simulink model "m_robotic_phase"  (R2021b)
settings: Solver=ode4  StartTime=0.0  StopTime=tf  FixedStep=0.01  RelTol=1e-3
values from neighbouring files (symbols this model uses):
  X_init = 3*(rand(2,1)-0.5)    [PD_phase_robotic.m]    (also in phase_robotic.m = 2*(rand(2,1)-0.5))
  Xd_init = 3*(rand(2,1)-0.5)    [PD_phase_robotic.m]    (also in phase_robotic.m = 1*(rand(2,1)-0.5))
settings Model: Creator=Mando  LastModifiedBy=Mando

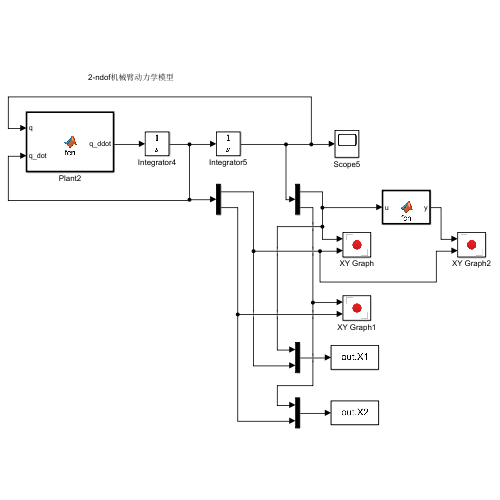
[thumbnail: Simulink's stored preview of the top-level diagram]
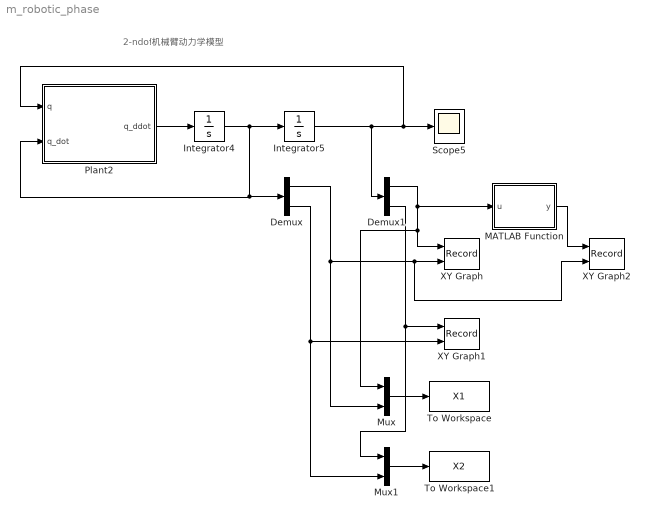
== system m_robotic_phase ==
  note: 2-ndof机械臂动力学模型
  Demux : Demux  Outputs=2
  Demux1 : Demux  Outputs=2
  Integrator4 : Integrator  InitialCondition=Xd_init
  Integrator5 : Integrator  InitialCondition=X_init
  MATLAB Function : MATLAB Function  TreatAsAtomicUnit=on
  Mux : Mux  Inputs=2
  Mux1 : Mux  Inputs=2
  Plant2 : MATLAB Function  TreatAsAtomicUnit=on
  Scope5 : Scope
  To Workspace : ToWorkspace  VariableName=X1  SampleTime=-1
  To Workspace1 : ToWorkspace  VariableName=X2  SampleTime=-1
  XY Graph : Record  FileSettingsInternal="{\"entries\":[{\"content\":{\"excelSettings\":{\"content\":{},\"type\":\"Streamout.ExcelSettings\"}},\"type\":\"Streamout.FileSettingStorage\",\"uuid\":\"9ba65a72-57f1-4f4d-8fe5-731dedb9ab80\"}],\"packageUris\":[\"http://schema.mathworks.com/mf0/streamout_blocks/R2020a\"],\"version\":\"1.0\"}"  Layout=[1 1]  SignalsInternal="{\"entries\":[{\"content\":{\"signals\":[{\"content\":{\"blockPath\":[\"m_robotic_phase/XY Graph\"],\"channel\":[],\"dimensions\":[1],\"domain\":\"m_robotic_phase/XY Graph\",\"lineColor\":\"#a2142f\",\"plots\":[1],\"port\":1,\"sid\":[\"\"],\"signalID\":74337,\"signalName\":\"Demux1:1\"},\"type\":\"RecordBlkView.Signal\",\"uuid\":\"b7ffe641-bfda-4282-85d4-15944fe21698\"},{\"content\":{\"blockPath\":[\"m_robotic_phase/XY Graph\"],\"channel\":[],\"dimensions\":[1],\"domain\":\"m_robotic_phase/XY Graph\",\"lineColor\":\"#139fff\",\"plots\":[1],\"port\":2,\"sid\":[\"\"],\"signalID\":74341,\"signalName\":\"Demux:1\"},\"type\":\"RecordBlkView.Signal\",\"uuid\":\"c2682a94-b715-47cb-b18e-efeff7ca8082\"}]},\"type\":\"RecordBlkView.InputSignals\",\"uuid\":\"df0cf377-e009-45f0-a3f5-9482d05fefdb\"}],\"packageUris\":[\"http://schema.mathworks.com/mf0/streamout_blocks/R2020a\"],\"version\":\"1.0\"}"  VisualizationBindings="{\"xyplotplugin\":{\"info\":[{\"series\":[{\"bindingParametersList\":[{\"parameter\":\"X-Axis\",\"signalID\":74337,\"signalName\":\"Demux1:1\"},{\"parameter\":\"Y-Axis\",\"signalID\":74341,\"signalName\":\"Demux:1\"}],\"seriesID\":17156}],\"subplotID\":1}]}}"  CompatibilityTag=XY
  XY Graph1 : Record  FileSettingsInternal="{\"entries\":[{\"content\":{\"excelSettings\":{\"content\":{},\"type\":\"Streamout.ExcelSettings\"}},\"type\":\"Streamout.FileSettingStorage\",\"uuid\":\"662d732d-d3fd-4f1e-9c42-ec22ce91c877\"}],\"packageUris\":[\"http://schema.mathworks.com/mf0/streamout_blocks/R2020a\"],\"version\":\"1.0\"}"  Layout=[1 1]  SignalsInternal="{\"entries\":[{\"content\":{\"signals\":[{\"content\":{\"blockPath\":[\"m_robotic_phase/XY Graph1\"],\"channel\":[],\"dimensions\":[1],\"domain\":\"m_robotic_phase/XY Graph1\",\"lineColor\":\"#a2142f\",\"plots\":[1],\"port\":1,\"sid\":[\"\"],\"signalID\":74345,\"signalName\":\"Demux1:2\"},\"type\":\"RecordBlkView.Signal\",\"uuid\":\"3157ee18-e9c7-4511-a6da-90271443b8bf\"},{\"content\":{\"blockPath\":[\"m_robotic_phase/XY Graph1\"],\"channel\":[],\"dimensions\":[1],\"domain\":\"m_robotic_phase/XY Graph1\",\"lineColor\":\"#139fff\",\"plots\":[1],\"port\":2,\"sid\":[\"\"],\"signalID\":74349,\"signalName\":\"Demux:2\"},\"type\":\"RecordBlkView.Signal\",\"uuid\":\"5d7954bb-a68d-4f60-a200-3899f2a7276c\"}]},\"type\":\"RecordBlkView.InputSignals\",\"uuid\":\"7aff9f94-aa5e-4cda-a56e-6b9542cacd60\"}],\"packageUris\":[\"http://schema.mathworks.com/mf0/streamout_blocks/R2020a\"],\"version\":\"1.0\"}"  VisualizationBindings="{\"xyplotplugin\":{\"info\":[{\"series\":[{\"bindingParametersList\":[{\"parameter\":\"X-Axis\",\"signalID\":74345,\"signalName\":\"Demux1:2\"},{\"parameter\":\"Y-Axis\",\"signalID\":74349,\"signalName\":\"Demux:2\"}],\"seriesID\":2777}],\"subplotID\":1}]}}"  CompatibilityTag=XY
  XY Graph2 : Record  FileSettingsInternal="{\"entries\":[{\"content\":{\"excelSettings\":{\"content\":{},\"type\":\"Streamout.ExcelSettings\"}},\"type\":\"Streamout.FileSettingStorage\",\"uuid\":\"226ea169-6c01-4002-94a1-aa70f380c900\"}],\"packageUris\":[\"http://schema.mathworks.com/mf0/streamout_blocks/R2020a\"],\"version\":\"1.0\"}"  Layout=[1 1]  SignalsInternal="{\"entries\":[{\"content\":{\"signals\":[{\"content\":{\"blockPath\":[\"m_robotic_phase/XY Graph2\"],\"channel\":[],\"dimensions\":[1],\"domain\":\"m_robotic_phase/XY Graph2\",\"lineColor\":\"#a2142f\",\"plots\":[1],\"port\":1,\"sid\":[\"\"],\"signalID\":74353,\"signalName\":\"MATLAB Function\"},\"type\":\"RecordBlkView.Signal\",\"uuid\":\"c744f4cf-835b-42c5-bc37-115fd98b61a8\"},{\"content\":{\"blockPath\":[\"m_robotic_phase/XY Graph2\"],\"channel\":[],\"dimensions\":[1],\"domain\":\"m_robotic_phase/XY Graph2\",\"lineColor\":\"#139fff\",\"plots\":[1],\"port\":2,\"sid\":[\"\"],\"signalID\":74357,\"signalName\":\"Demux:1\"},\"type\":\"RecordBlkView.Signal\",\"uuid\":\"48d42c33-c048-40b2-a4d2-4828affef8a8\"}]},\"type\":\"RecordBlkView.InputSignals\",\"uuid\":\"c4ee1b86-260e-4974-a977-5a9435b7889e\"}],\"packageUris\":[\"http://schema.mathworks.com/mf0/streamout_blocks/R2020a\"],\"version\":\"1.0\"}"  VisualizationBindings="{\"xyplotplugin\":{\"info\":[{\"series\":[{\"bindingParametersList\":[{\"parameter\":\"X-Axis\",\"signalID\":74353,\"signalName\":\"MATLAB Function\"},{\"parameter\":\"Y-Axis\",\"signalID\":74357,\"signalName\":\"Demux:1\"}],\"seriesID\":55931}],\"subplotID\":1}]}}"  CompatibilityTag=XY
  wires:
  Integrator5/1 -> Demux1/1, Plant2/1(q), Scope5/1
  Integrator4/1 -> Integrator5/1, Demux/1, Plant2/2(q_dot)
  Plant2/1(q_ddot) -> Integrator4/1
  Demux1/1 -> MATLAB Function/1(u), Mux/1, XY Graph/1
  Demux/1 -> XY Graph2/2, XY Graph/2, Mux/2
  Demux1/2 -> Mux1/1, XY Graph1/1
  Demux/2 -> Mux1/2, XY Graph1/2
  MATLAB Function/1(y) -> XY Graph2/1
  Mux/1 -> To Workspace/1
  Mux1/1 -> To Workspace1/1

== matlab function m_robotic_phase/Plant2 ==
  data: q_ddot output; q input; q_dot input
function q_ddot = fcn( q, q_dot)
%Defining given parameters
p1=2.9;
p2=0.76;
p3=0.87;
p4=3.04;
p5=0.87;
g=9.8;


%Defining Robot Dynamic Model
M = [p1+p2+2*p3*cos(q(2)),p2+p3*cos(q(2));p2+p3*cos(q(2)),p2];
Vm=[-p3*q_dot(2)*sin(q(2)) -p3*(q_dot(1)+q_dot(2))*sin(q(2)); p3*q_dot(1)*sin(q(2)) 0];
G= [p4*g*cos(q(1))+p5*g*cos(q(1)+q(2));p5*g*cos(q(1)+q(2))];

%Robot Dynamics
q_ddot = inv(M)*( - (Vm*q_dot) - G);

== matlab function m_robotic_phase/MATLAB Function ==
  data: u input; y output
function y = fcn(u)



if u>0
    y=mod(u,2*pi);
elseif u<0 
    y=mod(u,-2*pi);

else
    y=u;
end
